simulink model "vekt_shim"  (R2019a)
settings: Solver=ode4  StartTime=0.0  StopTime=2  FixedStep=1e-5  RelTol=1e-3
libraries: powerlib x4, simulink x3, powerlib_meascontrol x1
settings Model: Creator=Sozonov_AA  LastModifiedBy=Sozonov_AA
settings DataIOCC: SaveOutput=off  SaveTime=off
settings OptimizationCC: DefaultParameterBehavior=Inlined  InlineInvariantSignals=on  EnhancedBackFolding=on  PassReuseOutputArgsAs=Individual arguments  StateBitsets=on  DataBitsets=on  ZeroExternalMemoryAtStartup=off  ZeroInternalMemoryAtStartup=off  NoFixptDivByZeroProtection=on  EfficientFloat2IntCast=on  OptimizeBlockOrder=speed  DifferentSizesBufferReuse=on
settings DebuggingCC: ParameterTunabilityLossMsg=error
settings SFSimCC: MATLABDynamicMemAlloc=off
settings RTWCC: SystemTargetFile=ert.tlc  TemplateMakefile=ert_default_tmf  GenerateReport=on  RTWVerbose=off  IncludeHyperlinkInReport=on  LaunchReport=on  GenerateTraceInfo=on  GenerateTraceReport=on  GenerateTraceReportSl=on  GenerateTraceReportSf=on  GenerateTraceReportEml=on
settings CodeAppCC: ForceParamTrailComments=on  IgnoreCustomStorageClasses=off  OperatorAnnotations=on  SimulinkDataObjDesc=on  SFDataObjDesc=on  CustomSymbolStrGlobalVar=rt$N$M  CustomSymbolStrType=$N$M  CustomSymbolStrFcn=$N$M$F  CustomSymbolStrMacro=$N$M  InsertBlockDesc=on
settings ERTTargetCC: TargetLangStandard=C99 (ISO)  GenerateSampleERTMain=on  IncludeMdlTerminateFcn=off  CombineSignalStateStructs=on  PurelyIntegerCode=on  SupportNonFinite=off  InlinedParameterPlacement=NonHierarchical  ERTCustomFileTemplate=example_file_process.tlc

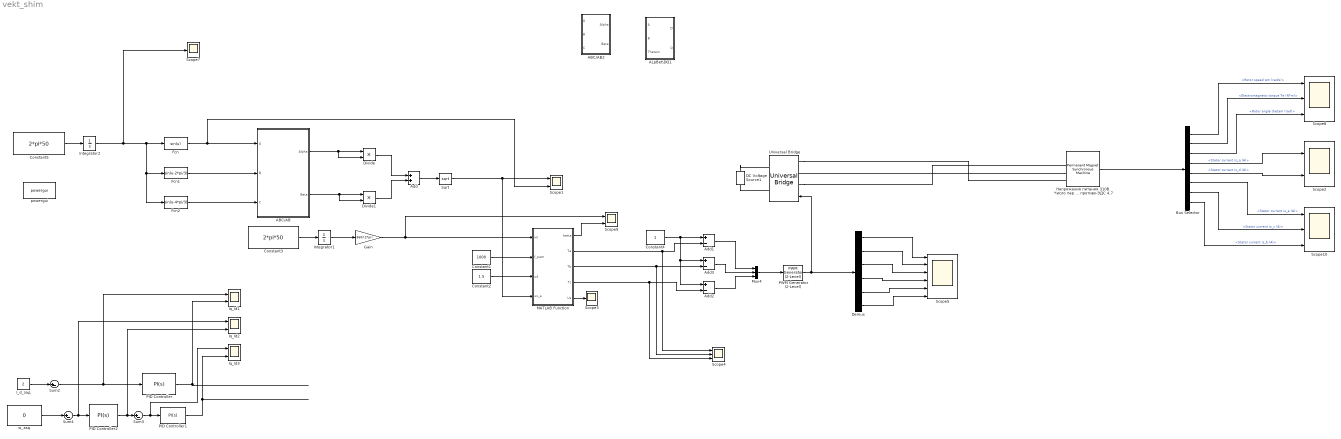
== system vekt_shim ==
  ABC/AB : Subsystem
  ABC/AB2 : Subsystem
  ALpBet\DQ1 : Subsystem
  Add : Sum
  Add1 : Sum  Inputs=+-
  Add2 : Sum  Inputs=+-
  Add3 : Sum  Inputs=+-
  Bus Selector : BusSelector  OutputSignals=Rotor speed wm (rad/s),Electromagnetic torque Te (N*m),Rotor angle thetam (rad),Stator current is_q (A),Stator current is_d (A),Stator current is_a (A),Stator current is_c (A),Stator current is_b (A)
  Constant1 : Constant  Value=1000
  Constant2 : Constant  Value=1.5
  Constant3 : Constant  Value=2*pi*50
  Constant4 : Constant
  Constant5 : Constant  Value=2*pi*50
  DC Voltage Source1 : powerlib/Electrical Sources/DC Voltage Source  Amplitude=310  Measurements=None
      settings: SourceProductName=Simscape Electrical
  Demux : Demux  Outputs=6
  Divide : Product  Inputs=**
  Divide1 : Product  Inputs=**
  Fcn : Fcn  Expr=sin(u)
  Fcn1 : Fcn  Expr=sin(u-2*pi/3)
  Fcn2 : Fcn  Expr=sin(u-4*pi/3)
  Gain : Gain  Gain=360/(2*pi)
  I_d_зад : Constant  Value=2
  Integrator1 : Integrator  InitialCondition=2*pi-pi/2  UpperSaturationLimit=2*pi  LowerSaturationLimit=0  WrapState=on  WrappedStateUpperValue=2*pi  WrappedStateLowerValue=0  ZeroCross=off
  Integrator2 : Integrator  UpperSaturationLimit=2*pi  LowerSaturationLimit=0  WrapState=on  WrappedStateUpperValue=2*pi  WrappedStateLowerValue=0  ZeroCross=off
  Iq_Id1 : Scope  NumInputPorts=2
  Iq_Id2 : Scope  NumInputPorts=2
  Iq_Id3 : Scope  NumInputPorts=2
  MATLAB Function : MATLAB Function  TreatAsAtomicUnit=on
  Mux4 : Mux  Inputs=3
  PID Controller : simulink/Continuous/PID Controller  Controller=PI  Form=Parallel  TimeDomain=Continuous-time  SampleTime=-1  IntegratorMethod=Forward Euler  FilterMethod=Forward Euler  ControllerParametersSource=internal  P=310*1.4142  I=20  D=0  UseFilter=on  N=100  TunerSelectOption=Transfer Function Based (PID Tuner App)  InitialConditionSource=internal  InitialConditionForIntegrator=0  InitialConditionForFilter=0  DifferentiatorICPrevScaledInput=0  ExternalReset=none  TrackingMode=off  Kt=1  LimitOutput=on  UpperSaturationLimit=1000  LowerSaturationLimit=-1000  LinearizeAsGain=on  AntiWindupMode=none  Kb=1  POutMin=[]  POutMax=[]  IOutMin=[]  IOutMax=[]  DOutMin=[]  DOutMax=[]  NOutMin=[]  NOutMax=[]  SumOutMin=[]  SumOutMax=[]  SaturationOutMin=[]  SaturationOutMax=[]  PParamMin=[]  PParamMax=[]  IParamMin=[]  IParamMax=[]  DParamMin=[]  DParamMax=[]  NParamMin=[]  NParamMax=[]  KbParamMin=[]  KbParamMax=[]  KtParamMin=[]  KtParamMax=[]  KbOutMin=[]  KbOutMax=[]  KtOutMin=[]  KtOutMax=[]  IntegratorOutMin=[]  IntegratorOutMax=[]  FilterOutMin=[]  FilterOutMax=[]  SumI1OutMin=[]  SumI1OutMax=[]  SumI2OutMin=[]  SumI2OutMax=[]  SumI3OutMin=[]  SumI3OutMax=[]  SumI4OutMin=[]  SumI4OutMax=[]  SumDOutMin=[]  SumDOutMax=[]  DifferentiatorOutMin=[]  DifferentiatorOutMax=[]  FilterDiffOutCoefMin=[]  FilterDiffOutCoefMax=[]  ReciprocalOutMin=[]  ReciprocalOutMax=[]  SumDenOutMin=[]  SumDenOutMax=[]  SumNumOutMin=[]  SumNumOutMax=[]  DivideOutMin=[]  DivideOutMax=[]  IntegratorContinuousStateAttributes=''  IntegratorStateMustResolveToSignalObject=off  IntegratorRTWStateStorageClass=Auto  FilterContinuousStateAttributes=''  FilterStateMustResolveToSignalObject=off  FilterRTWStateStorageClass=Auto  ParallelPVariant=InternalParameters  IdealPVariant=Disabled  IVariant=InternalParameters  DVariant=Disabled  IntegratorVariant=Continuous  SatVariant=Enabled  AWVariant=Passthrough  PCopyVariant=Disabled  TRVariant=Disabled  FdbkBlocksVariant=Forward  IdealPFdbkVariant=Disabled  SatFdbkVariant=Disabled  DerivativeFilterVariant=Disabled  NVariant=Disabled  NCopyVariant=Disabled_SignalSpec  FilterICVariant=Disabled  IntegratorICVariant=InternalICs  ExternalResetVariant=Disabled  TRSumVariant=Passthrough  SumFdbkVariant=Disabled  SumVariant=Sum_PI
  PID Controller1 : simulink/Continuous/PID Controller  Controller=PI  Form=Parallel  TimeDomain=Continuous-time  SampleTime=-1  IntegratorMethod=Forward Euler  FilterMethod=Forward Euler  ControllerParametersSource=internal  P=310*1.41/100  I=0.1  D=0  UseFilter=on  N=100  TunerSelectOption=Transfer Function Based (PID Tuner App)  InitialConditionSource=internal  InitialConditionForIntegrator=0  InitialConditionForFilter=0  DifferentiatorICPrevScaledInput=0  ExternalReset=none  TrackingMode=off  Kt=1  LimitOutput=on  UpperSaturationLimit=1000  LowerSaturationLimit=-1000  LinearizeAsGain=on  AntiWindupMode=none  Kb=1  POutMin=[]  POutMax=[]  IOutMin=[]  IOutMax=[]  DOutMin=[]  DOutMax=[]  NOutMin=[]  NOutMax=[]  SumOutMin=[]  SumOutMax=[]  SaturationOutMin=[]  SaturationOutMax=[]  PParamMin=[]  PParamMax=[]  IParamMin=[]  IParamMax=[]  DParamMin=[]  DParamMax=[]  NParamMin=[]  NParamMax=[]  KbParamMin=[]  KbParamMax=[]  KtParamMin=[]  KtParamMax=[]  KbOutMin=[]  KbOutMax=[]  KtOutMin=[]  KtOutMax=[]  IntegratorOutMin=[]  IntegratorOutMax=[]  FilterOutMin=[]  FilterOutMax=[]  SumI1OutMin=[]  SumI1OutMax=[]  SumI2OutMin=[]  SumI2OutMax=[]  SumI3OutMin=[]  SumI3OutMax=[]  SumI4OutMin=[]  SumI4OutMax=[]  SumDOutMin=[]  SumDOutMax=[]  DifferentiatorOutMin=[]  DifferentiatorOutMax=[]  FilterDiffOutCoefMin=[]  FilterDiffOutCoefMax=[]  ReciprocalOutMin=[]  ReciprocalOutMax=[]  SumDenOutMin=[]  SumDenOutMax=[]  SumNumOutMin=[]  SumNumOutMax=[]  DivideOutMin=[]  DivideOutMax=[]  IntegratorContinuousStateAttributes=''  IntegratorStateMustResolveToSignalObject=off  IntegratorRTWStateStorageClass=Auto  FilterContinuousStateAttributes=''  FilterStateMustResolveToSignalObject=off  FilterRTWStateStorageClass=Auto  ParallelPVariant=InternalParameters  IdealPVariant=Disabled  IVariant=InternalParameters  DVariant=Disabled  IntegratorVariant=Continuous  SatVariant=Enabled  AWVariant=Passthrough  PCopyVariant=Disabled  TRVariant=Disabled  FdbkBlocksVariant=Forward  IdealPFdbkVariant=Disabled  SatFdbkVariant=Disabled  DerivativeFilterVariant=Disabled  NVariant=Disabled  NCopyVariant=Disabled_SignalSpec  FilterICVariant=Disabled  IntegratorICVariant=InternalICs  ExternalResetVariant=Disabled  TRSumVariant=Passthrough  SumFdbkVariant=Disabled  SumVariant=Sum_PI
  PID Controller2 : simulink/Continuous/PID Controller  Controller=PI  Form=Parallel  TimeDomain=Continuous-time  SampleTime=-1  IntegratorMethod=Forward Euler  FilterMethod=Forward Euler  ControllerParametersSource=internal  P=100/533  I=0.1  D=0  UseFilter=on  N=100  TunerSelectOption=Transfer Function Based (PID Tuner App)  InitialConditionSource=internal  InitialConditionForIntegrator=0  InitialConditionForFilter=0  DifferentiatorICPrevScaledInput=0  ExternalReset=none  TrackingMode=off  Kt=1  LimitOutput=on  UpperSaturationLimit=1000  LowerSaturationLimit=-1000  LinearizeAsGain=on  AntiWindupMode=none  Kb=1  POutMin=[]  POutMax=[]  IOutMin=[]  IOutMax=[]  DOutMin=[]  DOutMax=[]  NOutMin=[]  NOutMax=[]  SumOutMin=[]  SumOutMax=[]  SaturationOutMin=[]  SaturationOutMax=[]  PParamMin=[]  PParamMax=[]  IParamMin=[]  IParamMax=[]  DParamMin=[]  DParamMax=[]  NParamMin=[]  NParamMax=[]  KbParamMin=[]  KbParamMax=[]  KtParamMin=[]  KtParamMax=[]  KbOutMin=[]  KbOutMax=[]  KtOutMin=[]  KtOutMax=[]  IntegratorOutMin=[]  IntegratorOutMax=[]  FilterOutMin=[]  FilterOutMax=[]  SumI1OutMin=[]  SumI1OutMax=[]  SumI2OutMin=[]  SumI2OutMax=[]  SumI3OutMin=[]  SumI3OutMax=[]  SumI4OutMin=[]  SumI4OutMax=[]  SumDOutMin=[]  SumDOutMax=[]  DifferentiatorOutMin=[]  DifferentiatorOutMax=[]  FilterDiffOutCoefMin=[]  FilterDiffOutCoefMax=[]  ReciprocalOutMin=[]  ReciprocalOutMax=[]  SumDenOutMin=[]  SumDenOutMax=[]  SumNumOutMin=[]  SumNumOutMax=[]  DivideOutMin=[]  DivideOutMax=[]  IntegratorContinuousStateAttributes=''  IntegratorStateMustResolveToSignalObject=off  IntegratorRTWStateStorageClass=Auto  FilterContinuousStateAttributes=''  FilterStateMustResolveToSignalObject=off  FilterRTWStateStorageClass=Auto  ParallelPVariant=InternalParameters  IdealPVariant=Disabled  IVariant=InternalParameters  DVariant=Disabled  IntegratorVariant=Continuous  SatVariant=Enabled  AWVariant=Passthrough  PCopyVariant=Disabled  TRVariant=Disabled  FdbkBlocksVariant=Forward  IdealPFdbkVariant=Disabled  SatFdbkVariant=Disabled  DerivativeFilterVariant=Disabled  NVariant=Disabled  NCopyVariant=Disabled_SignalSpec  FilterICVariant=Disabled  IntegratorICVariant=InternalICs  ExternalResetVariant=Disabled  TRSumVariant=Passthrough  SumFdbkVariant=Disabled  SumVariant=Sum_PI
  PWM Generator (2-Level) : powerlib_meascontrol/Pulse & Signal Generators/PWM Generator (2-Level)  ModulatorType=Three-phase bridge (6 pulses)  ModulatorMode=Unsynchronized  Fc=1000  Pc=90  nF=27  MinMax="[ 0  1 ]"  SamplingTechnique=Natural  ModulatingSignals=off  m=0.8  Freq=60  Phase=0  Ts=0  ShowCarrierOutport=off
  Scope1 : Scope  NumInputPorts=2
  Scope10 : Scope  NumInputPorts=3
  Scope2 : Scope  NumInputPorts=2
  Scope3 : Scope
  Scope4 : Scope  NumInputPorts=3
  Scope5 : Scope  NumInputPorts=6
  Scope7 : Scope
  Scope8 : Scope  NumInputPorts=3
  Scope9 : Scope  NumInputPorts=2
  Sqrt : Sqrt  SaturateOnIntegerOverflow=on
  Sum2 : Sum  Inputs=|+-
  Sum3 : Sum  Inputs=|+-
  Sum4 : Sum  Inputs=|+-
  Universal Bridge : powerlib/Power Electronics/Universal Bridge  Arms=3  SnubberResistance=1e5  SnubberCapacitance=inf  Device=IGBT / Diodes  Ron=1e-3  Lon=0  ForwardVoltages="[  0  0  ]"  ForwardVoltage=0  GTOparameters=[ 10e-6 , 20e-6 ]  IGBTparameters=[ 1e-6 , 2e-6 ]  Measurements=None  Measurements_2=None  converterType=Rectifier
      settings: SourceProductName=Simscape Electrical
  powergui : powerlib/powergui  Priority=1  SimulationMode=Continuous  SampleTime=50e-6  frequency=60  Iterations=50  frequencyindice=0  Pbase=100e6  ErrMax=1e-4  UnitsV=kV  UnitsW=MW  buscounter=0  FunctionMessages=off  echomessages=off  EnableUseOfTLC=off  CurrentSourceSwitches=off  DisableSnubberDevices=off  DisableRonSwitches=off  DisableVfSwitches=off  DisplayEquations=off  AutomaticDiscreteSolvers=off  SolverType=Tustin/Backward Euler (TBE)  Interpol=off  ExternalGateDelay=off  methode=off  Ts=100  x0status=blocks  SPID=on  SwTol=0  HookPort=off  NonlinearTolerance=0  nMaxIteration=15  ContinueOnMaxIteration=off  RestoreLinks=warning  ResistiveCurrentMeasurement=off  Frange=[0:2:500]  Ylog=off  Xlog=on  ShowGrid=off  save=off  variable=ZData  structure=0  ZoomFFT=off  StartTime=0.0  cycles=1  DisplayStyle=1  fundamental=60  FreqAxis=off  MaxFrequency=1000  frequencyindicesteady=1  RmsSteady=1  display=off
      settings: SourceProductName=Simscape Electrical
  "w_зад " : Constant  Value=0
  "Напряжения питания 310В. Число пар полюсов 10. Момент инерции ротора 0,003 кг/м2 . Длит. момент возд. охл. 19,5 Нм. Момент трения в подшипниках 1 Нм. Зубцовый момент 1 Нм. Максимальная скорость при Ma 444 об/мин. Скорость холостого хода при Mb 533 об/мин. Длит. ток с возд. охл. 3,4 А. Ток ХХ при Mb и Nb 0,7 А. КПД при Ma и Us 84,1%. Электрическое сопротивление при 20 град. Цельсия 5,92 Ом. Индуктивность 39,8 мГн. Коэффициент момента 5,7. Коэффициент противо-ЭДС 4,7 " : powerlib/Machines/Permanent Magnet Synchronous Machine  NbPhases=3  FluxDistribution=Sinusoidal  RotorType=Round  MechanicalLoad=Torque Tm  PresetModel=No  ShowDetailedParameters=on  MeasurementBus=off  Resistance=5.92  Inductance=8.5e-3  dqInductances=[8.5e-3,8.5e-3]  La=(39.8e-3)/2  MachineConstant=Torque Constant (N.m / A_peak)  Flux=0.38  VoltageCst=689.2438  TorqueCst=5.7  Flat=120  Mechanical=[0.003 0 10 0]  PolePairs=4  InitialConditions=[0,0, 0,0]  InitialConditions5ph=[0 0 0 0 0 0]  TsPowergui=0  TsBlock=-1  RefAngle=90 degrees behind phase A axis (modified Park)
  wires:
  Integrator2/1 -> Fcn/1, Fcn2/1, Fcn1/1, Scope7/1
  Constant5/1 -> Integrator2/1
  Gain/1 -> Scope9/1, MATLAB Function/1(wt)
  MATLAB Function/1(betta) -> Scope9/2
  Constant1/1 -> MATLAB Function/2(f_pwm)
  Constant2/1 -> MATLAB Function/3(ud)
  Fcn/1 -> Scope1/2, ABC/AB/1(A)
  Fcn1/1 -> ABC/AB/2(B)
  Fcn2/1 -> ABC/AB/3(C)
  ABC/AB/1(Alpha) -> Divide/2, Divide/1
  ABC/AB/2(Beta) -> Divide1/1, Divide1/2
  Add/1 -> Sqrt/1
  Divide/1 -> Add/1
  Divide1/1 -> Add/2
  Sqrt/1 -> MATLAB Function/4(us_a), Scope1/1
  MATLAB Function/2(Ta) -> Scope4/1, Add1/2
  MATLAB Function/3(Tb) -> Scope4/2, Add3/2
  MATLAB Function/4(Tc) -> Scope4/3, Add2/2
  MATLAB Function/5(Us) -> Scope3/1
  Constant3/1 -> Integrator1/1
  Integrator1/1 -> Gain/1
  Mux4/1 -> PWM Generator (2-Level)/1
  Constant4/1 -> Add2/1, Add3/1, Add1/1
  Add1/1 -> Mux4/1
  Add3/1 -> Mux4/2
  Add2/1 -> Mux4/3
  Demux/1 -> Scope5/1
  Demux/2 -> Scope5/2
  Demux/3 -> Scope5/3
  Demux/4 -> Scope5/4
  Demux/5 -> Scope5/5
  Demux/6 -> Scope5/6
  PWM Generator (2-Level)/1 -> Universal Bridge/1, Demux/1
  "Напряжения питания 310В. Число пар полюсов 10. Момент инерции ротора 0,003 кг/м2 . Длит. момент возд. охл. 19,5 Нм. Момент трения в подшипниках 1 Нм. Зубцовый момент 1 Нм. Максимальная скорость при Ma 444 об/мин. Скорость холостого хода при Mb 533 об/мин. Длит. ток с возд. охл. 3,4 А. Ток ХХ при Mb и Nb 0,7 А. КПД при Ma и Us 84,1%. Электрическое сопротивление при 20 град. Цельсия 5,92 Ом. Индуктивность 39,8 мГн. Коэффициент момента 5,7. Коэффициент противо-ЭДС 4,7 "/1 -> Bus Selector/1
  PID Controller/1 -> Iq_Id1/2
  Sum4/1 -> PID Controller2/1, Iq_Id2/1
  ? -> Sum2/2  "Id"
  I_d_зад/1 -> Sum2/1
  Sum3/1 -> Iq_Id3/1, PID Controller1/1
  PID Controller1/1 -> Iq_Id3/2
  Sum2/1 -> Iq_Id1/1, PID Controller/1
  "w_зад "/1 -> Sum4/1
  ? -> Sum4/2  "Nr"
  PID Controller2/1 -> Iq_Id2/2, Sum3/1
  ? -> Sum3/2  "Iq"
  Bus Selector/1 -> Scope8/1  "<Rotor speed wm (rad/s)>"
  Bus Selector/2 -> Scope8/2  "<Electromagnetic torque Te (N*m)>"
  Bus Selector/3 -> Scope8/3  "<Rotor angle thetam (rad)>"
  Bus Selector/4 -> Scope2/1  "<Stator current is_q (A)>"
  Bus Selector/5 -> Scope2/2  "<Stator current is_d (A)>"
  Bus Selector/6 -> Scope10/1  "<Stator current is_a (A)>"
  Bus Selector/7 -> Scope10/2  "<Stator current is_c (A)>"
  Bus Selector/8 -> Scope10/3  "<Stator current is_b (A)>"
  connections:
  Universal Bridge/LConn1 -- "Напряжения питания 310В. Число пар полюсов 10. Момент инерции ротора 0,003 кг/м2 . Длит. момент возд. охл. 19,5 Нм. Момент трения в подшипниках 1 Нм. Зубцовый момент 1 Нм. Максимальная скорость при Ma 444 об/мин. Скорость холостого хода при Mb 533 об/мин. Длит. ток с возд. охл. 3,4 А. Ток ХХ при Mb и Nb 0,7 А. КПД при Ma и Us 84,1%. Электрическое сопротивление при 20 град. Цельсия 5,92 Ом. Индуктивность 39,8 мГн. Коэффициент момента 5,7. Коэффициент противо-ЭДС 4,7 "/LConn1
  Universal Bridge/LConn3 -- "Напряжения питания 310В. Число пар полюсов 10. Момент инерции ротора 0,003 кг/м2 . Длит. момент возд. охл. 19,5 Нм. Момент трения в подшипниках 1 Нм. Зубцовый момент 1 Нм. Максимальная скорость при Ma 444 об/мин. Скорость холостого хода при Mb 533 об/мин. Длит. ток с возд. охл. 3,4 А. Ток ХХ при Mb и Nb 0,7 А. КПД при Ma и Us 84,1%. Электрическое сопротивление при 20 град. Цельсия 5,92 Ом. Индуктивность 39,8 мГн. Коэффициент момента 5,7. Коэффициент противо-ЭДС 4,7 "/LConn3
  "Напряжения питания 310В. Число пар полюсов 10. Момент инерции ротора 0,003 кг/м2 . Длит. момент возд. охл. 19,5 Нм. Момент трения в подшипниках 1 Нм. Зубцовый момент 1 Нм. Максимальная скорость при Ma 444 об/мин. Скорость холостого хода при Mb 533 об/мин. Длит. ток с возд. охл. 3,4 А. Ток ХХ при Mb и Nb 0,7 А. КПД при Ma и Us 84,1%. Электрическое сопротивление при 20 град. Цельсия 5,92 Ом. Индуктивность 39,8 мГн. Коэффициент момента 5,7. Коэффициент противо-ЭДС 4,7 "/LConn2 -- Universal Bridge/LConn2
  DC Voltage Source1/RConn1 -- Universal Bridge/RConn1
  DC Voltage Source1/LConn1 -- Universal Bridge/RConn2

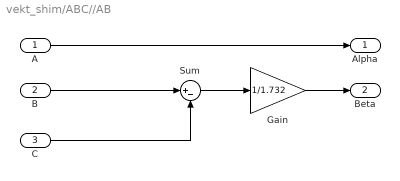
== system vekt_shim/ABC//AB ==
  A : Inport
  B : Inport  Port=2
  C : Inport  Port=3
  Gain : Gain  Gain=1/1.732
  Sum : Sum  Inputs=|+-
  Alpha : Outport
  Beta : Outport  Port=2
  wires:
  B/1 -> Sum/1
  C/1 -> Sum/2
  Sum/1 -> Gain/1
  A/1 -> Alpha/1
  Gain/1 -> Beta/1

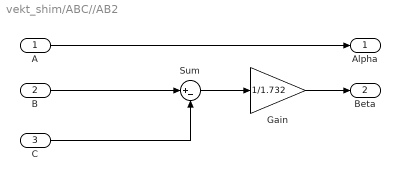
== system vekt_shim/ABC//AB2 ==
  A : Inport
  B : Inport  Port=2
  C : Inport  Port=3
  Gain : Gain  Gain=1/1.732
  Sum : Sum  Inputs=|+-
  Alpha : Outport
  Beta : Outport  Port=2
  wires:
  Gain/1 -> Beta/1
  A/1 -> Alpha/1
  Sum/1 -> Gain/1
  C/1 -> Sum/2
  B/1 -> Sum/1

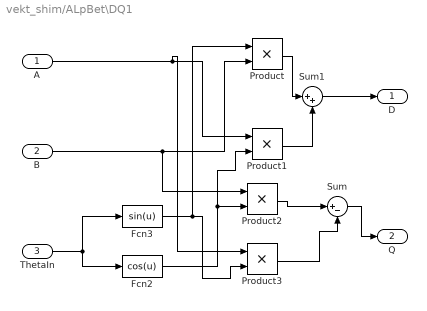
== system vekt_shim/ALpBet\DQ1 ==
  A : Inport
  B : Inport  Port=2
  ThetaIn : Inport  Port=3
  Fcn2 : Fcn  Expr=cos(u)
  Fcn3 : Fcn  Expr=sin(u)
  Product{,1..3} (4 alike) : Product  RndMeth=Zero
  Sum : Sum  Inputs=|+-
  Sum1 : Sum  Inputs=|++
  D : Outport
  Q : Outport  Port=2
  wires:
  Product3/1 -> Sum/2
  Product2/1 -> Sum/1
  Sum/1 -> Q/1
  Sum1/1 -> D/1
  Product1/1 -> Sum1/2
  Product/1 -> Sum1/1
  A/1 -> Product3/1, Product1/1
  Fcn2/1 -> Product2/2, Product1/2
  Fcn3/1 -> Product3/2, Product/1
  B/1 -> Product2/1, Product/2
  ThetaIn/1 -> Fcn2/1, Fcn3/1

== matlab function vekt_shim/MATLAB Function ==
  data: wt input; betta output; f_pwm input; ud input; us_a input; Ta output; Tb output; Tc output; Us output
function [ betta, Ta, Tb, Tc, Us] = fcn(wt, f_pwm, ud, us_a)
a_h=0;
b_h=0;
c_h=0;
a_l=0;
b_l=0;
c_l=0;
v=0;
t_pwm = (1/f_pwm);
Us = sqrt(3)*us_a/ud;


if (wt >= 0 && wt < 60)%базовый вектор 1
    v=1;
end    
if (wt > 60 && wt < 120)%базовый вектор 2
    v=2;
end
if (wt > 120 && wt < 180)%базовый вектор 3
    v=3;  
end
if (wt > 180 && wt < 240)%базовый вектор 4
    v=4; 
end
if (wt > 240 && wt < 300)%базовый вектор 5
    v=5; 
end
if (wt > 300 && wt <= 360)%базовый вектор 6
    v=6;      
end
   
betta=60-(v*60-wt);

T_1=Us*sin((60-betta)*2*pi/360);
T_2=Us*sin((betta)*2*pi/360);
T_0=1-T_1-T_2;

t_1=T_1+T_2+(T_0/2);
t_2=T_2+(T_0/2);
t_3=T_1+(T_0/2);
Ta=0;
Tb=0;
Tc=0;

if(v==1)
    Ta=t_1;
    Tb=t_2;
    Tc=T_0/2;
end    
if(v==2)
    Ta=t_3;
    Tb=t_1;
    Tc=T_0/2;
end
if(v==3)
    Ta=T_0/2;
    Tb=t_1;
    Tc=t_2;
end
if(v==4)
    Ta=T_0/2;
    Tb=t_3;
    Tc=t_1;
end
if(v==5)
    Ta=t_2;
    Tb=T_0/2;
    Tc=t_1;
end
if(v==6)
    Ta=t_1;
    Tb=T_0/2;
    Tc=t_3;
end
